simulink model "extra_stap_blocks"  (R2022a)
settings: Solver=VariableStepAuto  StartTime=0.0  StopTime=10.0  RelTol=1e-3
undefined symbols (not defined in the file or in its folder): paramSTAP
settings Model: Creator=frconway  LastModifiedBy=frconway

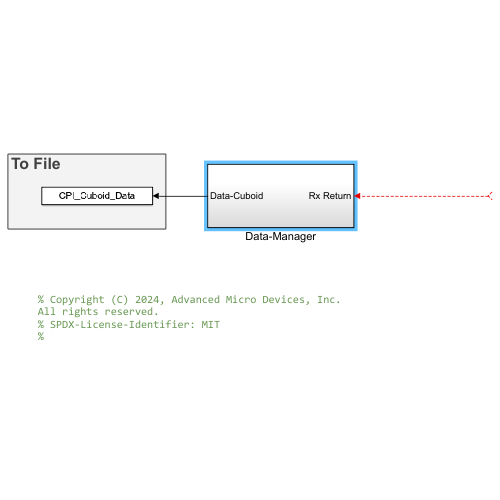
[thumbnail: Simulink's stored preview of the top-level diagram]
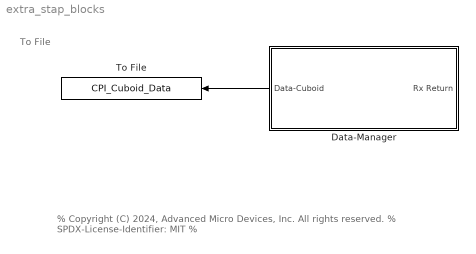
== system extra_stap_blocks ==
  note: To File
  note: % Copyright (C) 2024, Advanced Micro Devices, Inc. All rights reserved.
      | % SPDX-License-Identifier: MIT
      | %
  Data-Manager : Subsystem
  To File : ToFile  Filename=CPI_Cuboid_Data  MatrixName=Cuboid  SaveFormat=Timeseries
  wires:
  ? -> Data-Manager/1(Rx Return)
  Data-Manager/1(Data-Cuboid) -> To File/1

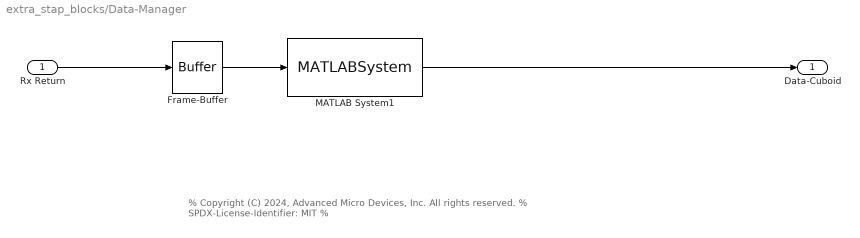
== system extra_stap_blocks/Data-Manager ==
  note: % Copyright (C) 2024, Advanced Micro Devices, Inc. All rights reserved.
      | % SPDX-License-Identifier: MIT
      | %
  Rx Return : Inport
  Frame-Buffer : Buffer  N=paramSTAP.numPulseInt*(paramSTAP.samplesPerFrame)  ic=eps*randn(2*paramSTAP.numPulseInt*(paramSTAP.samplesPerFrame),paramSTAP.radarAntenna.NumElements)
  MATLAB System1 : MATLABSystem  System=phased.internal.MatrixCubeConverter  NumPages=paramSTAP.numPulseInt  SimulateUsing=Interpreted execution
      mask Type: phased.internal.MatrixCubeConverter
      mask Display:
      | disp('Matrix -> Cube');
      | port_label('input',1,'X');
      | port_label('output',1,'XC');
  Data-Cuboid : Outport
  wires:
  Frame-Buffer/1 -> MATLAB System1/1
  MATLAB System1/1 -> Data-Cuboid/1
  Rx Return/1 -> Frame-Buffer/1
